simulink model "simli_gridSI"  (R2023b)
settings: Solver=VariableStepAuto  StartTime=0.0  StopTime=20  RelTol=1e-3
undefined symbols (not defined in the file or in its folder): c_f, Cbase1v, delta_vsc_0, G_dc_denom, G_dc_num, H_gen, H_vsm, Ibase_lv, k_d_vsm, k_p_p_vsm, k_p_q_vsm, ki_q, ki_vc, kp_vc, l_f, Lbase1v, M_gr_denom, M_gr_num, mppt_gain, omega_nom, omega_WTR_0, omega_WTR_n, P_aero_0, P_meas, Q_meas, r_f, r_grid, Rd, T_dc_denom, T_dc_num, Ts_power, v_D_t, v_Q_t, Vbase_lv, vect, x_sys, Zbase1v
libraries: slpidlib x2, spspowerguiLib x1
settings Model: Creator=Martin Pedersen  LastModifiedBy=marti

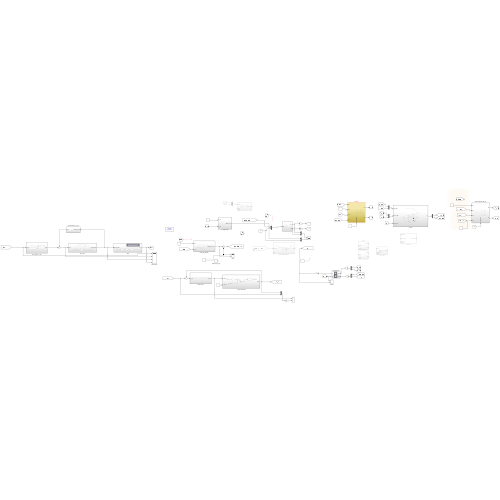
[thumbnail: Simulink's stored preview of the top-level diagram]
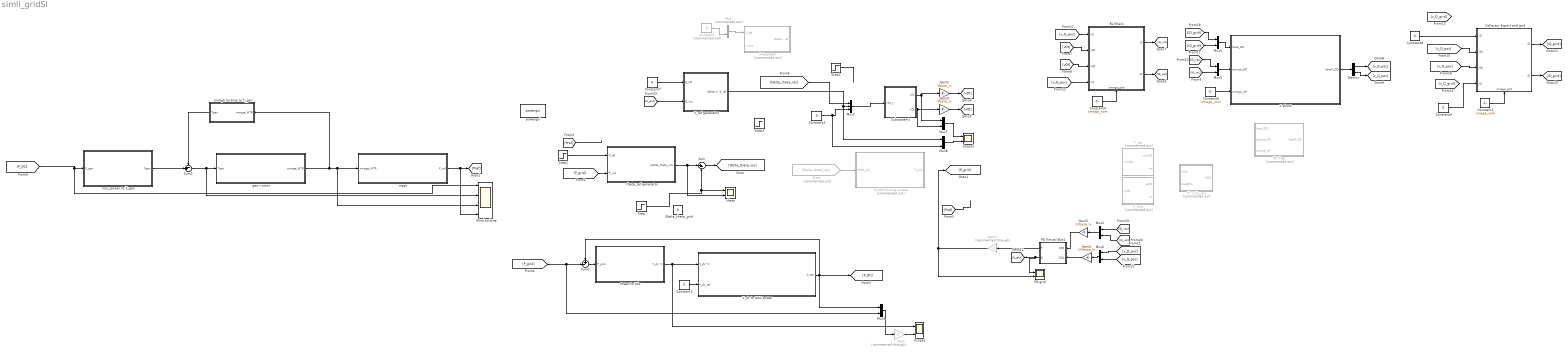
== system simli_gridSI ==
  C shunt : Subsystem
  Collector Export and grid : Subsystem
      settings: PortSchema="{\"entries\":[{\"content\":{\"sides\":[{\"content\":{\"connectorIds\":[\"In1\",\"In2\",\"In3\",\"In4\"]},\"type\":\"ConnectorPlacement.EquallySpacedRectSide\",\"uuid\":\"57ad71d1-5664-4b35-a20c-d71f7e1cdc47\"},{\"content\":{\"connectorIds\":[\"Out1\",\"Out2\"],\"side\":\"RIGHT\"},\"type\":\"ConnectorPlacement.EquallySpacedRectSide\",\"uuid\":\"8101605d-eedb-4c26-847d-0cc0ce629d60\"},{\"content\":{\"side\":\"TOP\"},\"type\":\"ConnectorPlacement.EquallySpacedRectSide\",\"uuid\":\"2627b00b-24a5-469a-be2d-9c3c8a1d2080\"},{\"content\":{\"connectorIds\":[\"In5\"],\"side\":\"BOTTOM\"},\"type\":\"ConnectorPlacement.EquallySpacedRectSide\",\"uuid\":\"fe553db7-7727-4a02-b1e7-5aedfb7840ee\"}]},\"type\":\"ConnectorPlacement.EquallySpacedConnector\",\"uuid\":\"f40200c8-ad5b-428c-8a4e-7641595b86c4\"}],\"packageUris\":[\"http://schema.mathworks.com/mf0/Connector/R2020b\"],\"version\":\"1.0\"}"
  Constant : Constant  Commented=on  Value=0
  Constant{1,3,7..9} (5 alike) : Constant  Value=0
  Constant2 : Constant  Value=omega_nom
  Constant4 : Constant  Value=omega_nom
  Constant5 : Constant  Value=omega_nom
  Demux : Demux  Outputs=2
  From : From  Commented=on  GotoTag=Delta_theta_vsc
  Gain : Gain  Commented=through  Gain=-1
  Gain1 : Gain  Commented=through  Gain=-1
  Gain2 : Gain  Gain=Vbase_lv
  Gain3 : Gain  Gain=Vbase_lv
  Gain4 : Gain  Gain=1/Vbase_lv
  Gain5 : Gain  Gain=1/Ibase_lv
  Mux : Mux  Commented=on  Inputs=2
  Mux{1,3..8} (7 alike) : Mux  Inputs=2
  Mux2 : Mux  Inputs=3
  PQ Virtual Bus1 : Subsystem
  PQ grid : Scope  NumInputPorts=2
  Power to Vdc : Subsystem
  RC filter : Subsystem  Commented=on  mask{Csource=c_f/omega_nom, Rd=0, VD0=1, VQ0=0}
      mask prompts: Csource "Net Capacitance"; Rd "Rdamp"
      mask help:
      | PI network, capacitance to enter is total.
      | Left and right current as input. Left and right voltage as output
      mask init:
      | inv_Csource=1/Csource;
      mask TypeOptions Csource: 8/Gain
      mask TypeOptions Rd: 1/Gain | 2/Gain
      mask TypeOptions VD0: VcpdR_int/InitialCondition
      mask TypeOptions VQ0: VcpqR_int/InitialCondition
  RL filter1 : Subsystem
      settings: PortSchema="{\"entries\":[{\"content\":{\"sides\":[{\"content\":{\"connectorIds\":[\"In1\",\"In2\",\"In3\",\"In4\"]},\"type\":\"ConnectorPlacement.EquallySpacedRectSide\",\"uuid\":\"57ad71d1-5664-4b35-a20c-d71f7e1cdc47\"},{\"content\":{\"connectorIds\":[\"Out1\",\"Out2\"],\"side\":\"RIGHT\"},\"type\":\"ConnectorPlacement.EquallySpacedRectSide\",\"uuid\":\"8101605d-eedb-4c26-847d-0cc0ce629d60\"},{\"content\":{\"side\":\"TOP\"},\"type\":\"ConnectorPlacement.EquallySpacedRectSide\",\"uuid\":\"2627b00b-24a5-469a-be2d-9c3c8a1d2080\"},{\"content\":{\"connectorIds\":[\"In5\"],\"side\":\"BOTTOM\"},\"type\":\"ConnectorPlacement.EquallySpacedRectSide\",\"uuid\":\"fe553db7-7727-4a02-b1e7-5aedfb7840ee\"}]},\"type\":\"ConnectorPlacement.EquallySpacedConnector\",\"uuid\":\"f40200c8-ad5b-428c-8a4e-7641595b86c4\"}],\"packageUris\":[\"http://schema.mathworks.com/mf0/Connector/R2020b\"],\"version\":\"1.0\"}"
  Scope1 : Scope  NumInputPorts=2
  Scope2 : Scope  NumInputPorts=2
  Step : Step  After=0.04  SampleTime=Ts_power
  Step1 : Step  After=0  SampleTime=Ts_power
  Step2 : Step  Time=5  After=0  SampleTime=Ts_power
  Step3 : Step  Time=5  After=0  SampleTime=Ts_power
  Subsystem : Subsystem  Commented=on
  Subsystem1 : Subsystem
  Sum : Sum  Inputs=|+-
  Sum1 : Sum  Inputs=+-|
  Sum2 : Sum  Inputs=-+|
  Synchronizing torque : Subsystem  Commented=on
  "T^{-1}_vsc" : Subsystem  Commented=on
  T_vsc : Subsystem  Commented=on  AncestorBlock=powerlib_meascontrol/Transformations/dq0 to Alpha-Beta-Zero/Subsystem1
  T_vsc1 : Subsystem  Commented=on  AncestorBlock=powerlib_meascontrol/Transformations/dq0 to Alpha-Beta-Zero/Subsystem1
  V_dc to MSC power : Subsystem
  V_ref generator : Subsystem
  Wind turbine : Scope  NumInputPorts=4
  \Delta_theta_grid : Constant  Value=0
  gen->rotor : Subsystem
  mppt : Subsystem
  msc_power to T_gen : Subsystem
  omega turbine to T_gen : Subsystem
  powergui : spspowerguiLib/powergui  Priority=1  SimulationMode=Discrete  SampleTime=Ts_power  frequency=60  Iterations=50  frequencyindice=60  Pbase=100e6  ErrMax=1e-4  UnitsV=kV  UnitsW=MW  buscounter=0  FunctionMessages=off  echomessages=off  EnableUseOfTLC=off  CurrentSourceSwitches=off  DisableSnubberDevices=off  DisableRonSwitches=off  DisableVfSwitches=off  DisplayEquations=off  AutomaticDiscreteSolvers=off  SolverType=Tustin/Backward Euler (TBE)  Interpol=off  ExternalGateDelay=off  methode=off  Ts=100  x0status=blocks  SPID=on  SwTol=0  HookPort=off  NonlinearTolerance=1e-4  nMaxIteration=100  ContinueOnMaxIteration=off  RestoreLinks=warning  ResistiveCurrentMeasurement=off  Frange=[0:2:500]  Ylog=off  Xlog=on  ShowGrid=off  save=off  variable=ZData  structure=0  ZoomFFT=off  StartTime=0.0  cycles=1  DisplayStyle=1  fundamental=60  FreqAxis=off  MaxFrequency=1000  frequencyindicesteady=1  RmsSteady=1  display=off
  theta : Scope  NumInputPorts=2
  theta_ref generator : Subsystem
  wires:
  theta_ref generator/1(\Delta_theta_vsm) -> theta/2, Sum/1
  Step/1 -> theta/1, Sum/2
  Sum/1 -> [Delta_theta_vsc]
  V_ref generator/1(\Delta V^d_ref) -> Mux8/1, Mux2/2
  Mux/1 -> Subsystem/1(V_ref)
  Constant/1 -> Mux/2
  From/1 -> Synchronizing torque/1(delta_vsc)
  PQ Virtual Bus1/1(P) -> Gain1/1
  [P_grid] -> theta_ref generator/2(P_vsc)
  [Pref] -> ?
  [Pref] -> ?
  gen->rotor/1(omega_WTR) -> omega turbine to T_gen/1(omega_WTR), Wind turbine/3, mppt/1(omega_WTR)
  Power to Vdc/1(V_dc^2) -> V_dc to MSC power/1(V_dc^2), Scope1/1
  V_dc to MSC power/1(P_DC) -> Mux1/1, [P_DC], Sum1/1
  Sum1/1 -> Power to Vdc/1(P_grid)
  [P_grid] -> Mux1/2, Sum1/2
  Mux1/1 -> Gain/1
  Sum2/1 -> Wind turbine/2, gen->rotor/1(Tgen)
  msc_power to T_gen/1(Tgen) -> Sum2/2
  omega turbine to T_gen/1(Tgen) -> Sum2/1
  [P_DC] -> Wind turbine/1, msc_power to T_gen/1(P_gen)
  mppt/1(P_ref) -> Wind turbine/4, [Pref]
  Constant1/1 -> V_dc to MSC power/2(V_dc_ref)
  Step1/1 -> theta_ref generator/1(P_ref)
  Gain/1 -> Scope1/2
  Constant3/1 -> Mux8/2, Mux2/3
  Step2/1 -> ?
  Mux2/1 -> Subsystem1/1(vdq_t)
  Constant4/1 -> RL filter1/5(omega_grid)
  Subsystem1/1(vDt) -> Mux7/1, Gain2/1
  Subsystem1/2(vQt) -> Mux7/2, Gain3/1
  [vDt] -> RL filter1/2(vDt)
  [vQt] -> RL filter1/3(vQt)
  Constant5/1 -> C shunt/3(omega_ref)
  RL filter1/2(iD) -> [iD_vsc]
  RL filter1/1(iQ) -> [iQ_vsc]
  Mux3/1 -> C shunt/2("Isource_DQ ")
  [iQ_vsc] -> Mux3/2
  [iD_vsc] -> Mux3/1
  C shunt/1(VpccR_DQ) -> Demux/1
  Demux/1 -> [v_D_poc]
  Demux/2 -> [v_Q_poc]
  [v_D_poc] -> RL filter1/1(vD)
  [v_Q_poc] -> RL filter1/4(vQ)
  Constant9/1 -> Collector Export and grid/4(vQ)
  Constant8/1 -> Collector Export and grid/1(vD)
  Collector Export and grid/1(iQ) -> [iQ_grid]
  Collector Export and grid/2(iD) -> [iD_grid]
  [v_Q_poc] -> Collector Export and grid/3(vQt)
  [v_D_poc] -> Collector Export and grid/2(vDt)
  Constant2/1 -> Collector Export and grid/5(omega_grid)
  Mux4/1 -> C shunt/1(Iload_DQ)
  [iQ_grid] -> Mux4/2
  [iD_grid] -> Mux4/1
  [iQ_vsc] -> Mux5/2
  [iD_vsc] -> Mux5/1
  Mux5/1 -> Gain5/1
  [v_Q_poc] -> Mux6/2
  [v_D_poc] -> Mux6/1
  Mux6/1 -> Gain4/1
  PQ Virtual Bus1/2(Q) -> PQ grid/1, [Q_grid]
  [Q_grid] -> V_ref generator/2(Q_vsc)
  Constant7/1 -> V_ref generator/1(Q_ref)
  Mux7/1 -> Scope2/1
  Mux8/1 -> Scope2/2
  [Delta_theta_vsc] -> Mux2/1
  Gain1/1 -> [P_grid], PQ grid/2
  Gain2/1 -> [vDt]
  Gain3/1 -> [vQt]
  Gain4/1 -> PQ Virtual Bus1/2(VDQ)
  Gain5/1 -> PQ Virtual Bus1/1(IDQ)

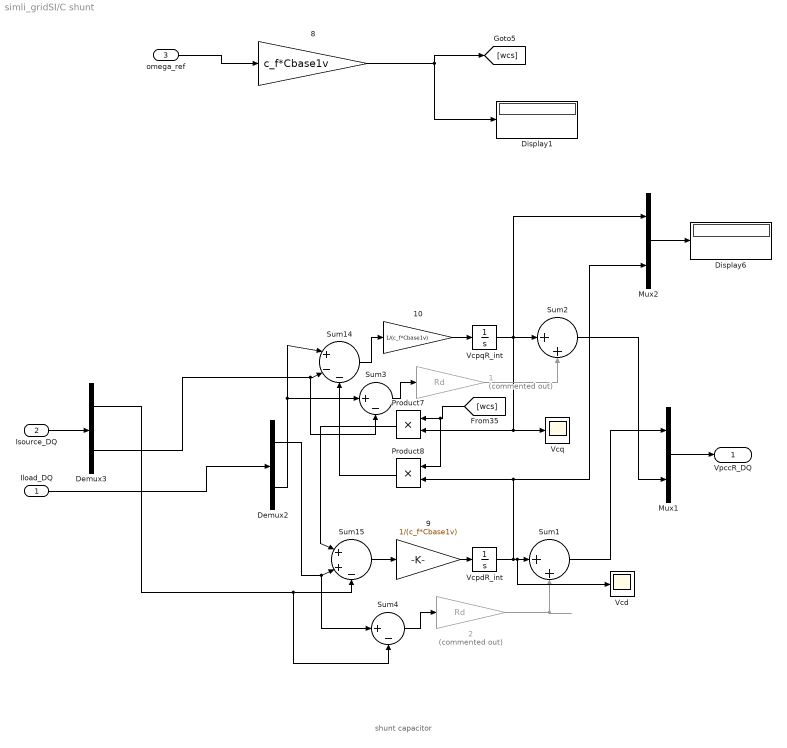
== system simli_gridSI/C shunt ==
  note: shunt capacitor
  Iload_DQ : Inport
  "Isource_DQ " : Inport  Port=2
  omega_ref : Inport  Port=3
  1 : Gain  Commented=on  Gain=Rd
  10 : Gain  Gain=1/(c_f*Cbase1v)
  2 : Gain  Commented=on  Gain=Rd
  8 : Gain  Gain=c_f*Cbase1v
  9 : Gain  Gain=1/(c_f*Cbase1v)
  Demux2 : Demux  Outputs=2
  Demux3 : Demux  Outputs=2
  Display1 : Display
  Display6 : Display
  Mux1 : Mux  Inputs=2
  Mux2 : Mux  Inputs=2
  Product7 : Product
  Product8 : Product
  Sum1 : Sum  Inputs=|++
  Sum14 : Sum  Inputs=|+--
  Sum15 : Sum  Inputs=|++-
  Sum2 : Sum  Inputs=|++
  Sum3 : Sum  Inputs=|+-
  Sum4 : Sum  Inputs=|+-
  Vcd : Scope
  VcpdR_int : Integrator  UpperSaturationLimit=50  LowerSaturationLimit=-1000
  VcpqR_int : Integrator  UpperSaturationLimit=50  LowerSaturationLimit=-1000
  Vcq : Scope
  VpccR_DQ : Outport  VectorParamsAs1DForOutWhenUnconnected=off
  wires:
  Mux1/1 -> VpccR_DQ/1
  Demux2/1 -> Sum15/2, Sum4/1
  VcpqR_int/1 -> Vcq/1, Product7/2, Sum2/1, Mux2/1
  1/1 -> Sum2/2
  2/1 -> Sum1/2
  Sum15/1 -> 9/1
  Product8/1 -> Sum14/3
  Sum14/1 -> 10/1
  8/1 -> [wcs], Display1/1
  Demux3/1 -> Sum15/3, Sum4/2
  "Isource_DQ "/1 -> Demux3/1
  Product7/1 -> Sum15/1
  omega_ref/1 -> 8/1
  Demux2/2 -> Sum14/1, Sum3/1
  [wcs] -> Product8/1, Product7/1
  Iload_DQ/1 -> Demux2/1
  9/1 -> VcpdR_int/1
  Demux3/2 -> Sum14/2, Sum3/2
  Sum3/1 -> 1/1
  10/1 -> VcpqR_int/1
  Mux2/1 -> Display6/1
  Sum4/1 -> 2/1
  Sum1/1 -> Mux1/1
  Sum2/1 -> Mux1/2
  VcpdR_int/1 -> Vcd/1, Sum1/1, Product8/2, Mux2/2

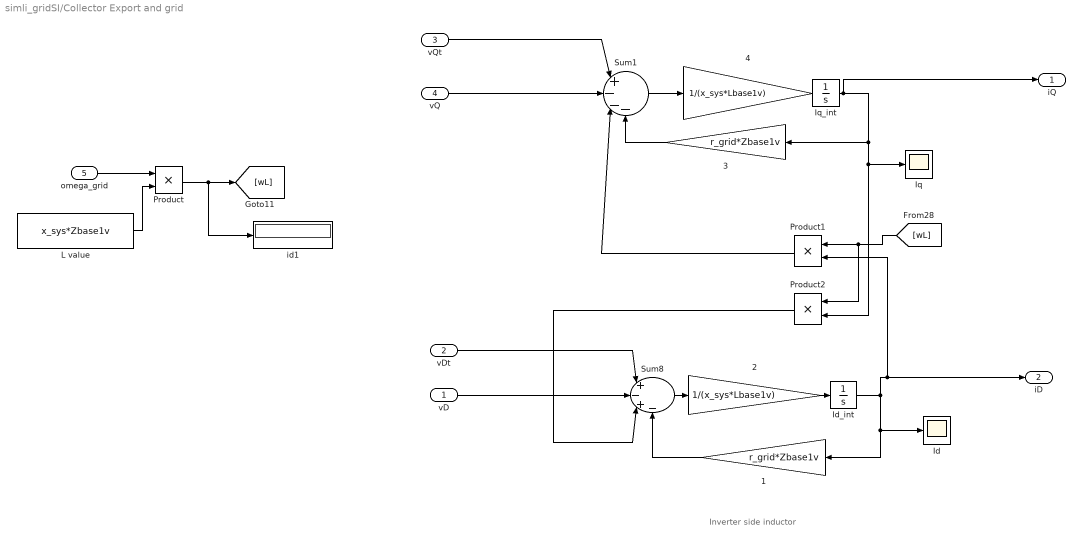
== system simli_gridSI/Collector Export and grid ==
  note: Inverter side inductor
  vD : Inport
  vDt : Inport  Port=2
  vQt : Inport  Port=3
  vQ : Inport  Port=4
  omega_grid : Inport  Port=5
  1 : Gain  Gain=r_grid*Zbase1v
  2 : Gain  Gain=1/(x_sys*Lbase1v)
  3 : Gain  Gain=r_grid*Zbase1v
  4 : Gain  Gain=1/(x_sys*Lbase1v)
  Id : Scope
  Id_int : Integrator  UpperSaturationLimit=50  LowerSaturationLimit=-1000
  Iq : Scope
  Iq_int : Integrator  UpperSaturationLimit=50  LowerSaturationLimit=-1000
  L value : Constant  Value=x_sys*Zbase1v  SampleTime=-1
  Product : Product
  Product1 : Product
  Product2 : Product
  Sum1 : Sum  Inputs=|+---
  Sum8 : Sum  Inputs=|+-+-
  id1 : Display
  iQ : Outport
  iD : Outport  Port=2
  wires:
  [wL] -> Product2/1, Product1/1
  Id_int/1 -> 1/1, Id/1, iD/1, Product1/2
  1/1 -> Sum8/4
  Product1/1 -> Sum1/3
  3/1 -> Sum1/4
  Sum1/1 -> 4/1
  2/1 -> Id_int/1
  Sum8/1 -> 2/1
  4/1 -> Iq_int/1
  Iq_int/1 -> iQ/1, Product2/2, Iq/1, 3/1
  Product2/1 -> Sum8/3
  vDt/1 -> Sum8/1
  vD/1 -> Sum8/2
  vQt/1 -> Sum1/1
  vQ/1 -> Sum1/2
  L value/1 -> Product/2
  Product/1 -> id1/1, [wL]
  omega_grid/1 -> Product/1

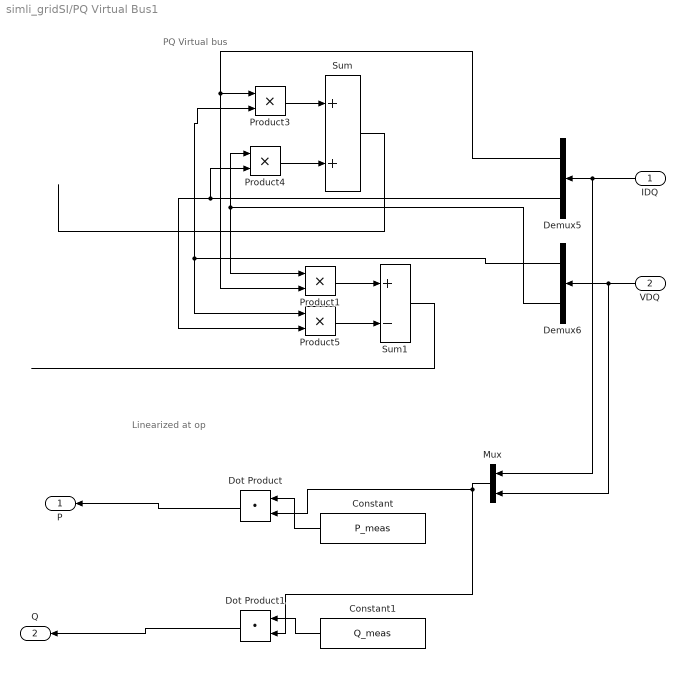
== system simli_gridSI/PQ Virtual Bus1 ==
  note: Linearized at op
  note: PQ Virtual bus
  IDQ : Inport
  VDQ : Inport  Port=2
  Constant : Constant  Value=P_meas
  Constant1 : Constant  Value=Q_meas
  Demux5 : Demux  Outputs=[vect vect]
  Demux6 : Demux  Outputs=[vect vect]
  Dot Product : DotProduct  OutDataTypeStr=Inherit: Inherit via internal rule
  Dot Product1 : DotProduct  OutDataTypeStr=Inherit: Inherit via internal rule
  Mux : Mux  Inputs=2
  Product{1,3..5} (4 alike) : Product  InputSameDT=on  SaturateOnIntegerOverflow=on  OutDataTypeStr=Inherit: Same as first input
  Sum : Sum  InputSameDT=on  SaturateOnIntegerOverflow=on  OutDataTypeStr=Inherit: Same as first input
  Sum1 : Sum  Inputs=+-  InputSameDT=on  SaturateOnIntegerOverflow=on  OutDataTypeStr=Inherit: Same as first input
  P : Outport
  Q : Outport  Port=2
  wires:
  Sum/1 -> ?
  VDQ/1 -> Mux/2, Demux6/1
  IDQ/1 -> Mux/1, Demux5/1
  Sum1/1 -> ?
  Product5/1 -> Sum1/2
  Product1/1 -> Sum1/1
  Demux6/2 -> Product4/1, Product1/1
  Demux5/1 -> Product1/2, Product3/1
  Demux6/1 -> Product3/2, Product5/1
  Product4/1 -> Sum/2
  Demux5/2 -> Product5/2, Product4/2
  Product3/1 -> Sum/1
  Constant/1 -> Dot Product/1
  Mux/1 -> Dot Product1/2, Dot Product/2
  Constant1/1 -> Dot Product1/1
  Dot Product1/1 -> Q/1
  Dot Product/1 -> P/1

== system simli_gridSI/Power to Vdc ==
  P_grid : Inport
  DC dynamics : TransferFcn  Numerator=T_dc_num{1}  Denominator=T_dc_denom{1}
  msc current control : TransferFcn  Commented=through  Denominator=[0.01 1]
  V_dc^2 : Outport
  wires:
  P_grid/1 -> msc current control/1
  DC dynamics/1 -> V_dc^2/1
  msc current control/1 -> DC dynamics/1

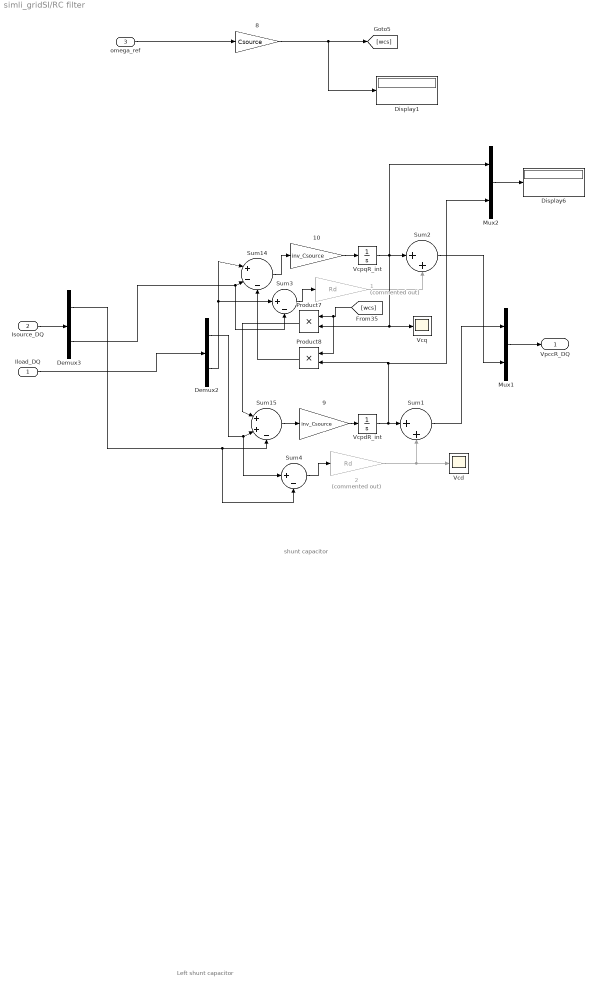
== system simli_gridSI/RC filter ==
  note: shunt capacitor
  note: Left shunt capacitor
  Iload_DQ : Inport
  "Isource_DQ " : Inport  Port=2
  omega_ref : Inport  Port=3
  1 : Gain  Commented=on  Gain=Rd
  10 : Gain  Gain=inv_Csource
  2 : Gain  Commented=on  Gain=Rd
  8 : Gain  Gain=Csource
  9 : Gain  Gain=inv_Csource
  Demux2 : Demux  Outputs=2
  Demux3 : Demux  Outputs=2
  Display1 : Display
  Display6 : Display
  Mux1 : Mux  Inputs=2
  Mux2 : Mux  Inputs=2
  Product7 : Product
  Product8 : Product
  Sum1 : Sum  Inputs=|++
  Sum14 : Sum  Inputs=|+--
  Sum15 : Sum  Inputs=|++-
  Sum2 : Sum  Inputs=|++
  Sum3 : Sum  Inputs=|+-
  Sum4 : Sum  Inputs=|+-
  Vcd : Scope
  VcpdR_int : Integrator  InitialCondition=VD0  UpperSaturationLimit=50  LowerSaturationLimit=-1000
  VcpqR_int : Integrator  InitialCondition=VQ0  UpperSaturationLimit=50  LowerSaturationLimit=-1000
  Vcq : Scope
  VpccR_DQ : Outport  VectorParamsAs1DForOutWhenUnconnected=off
  wires:
  Sum4/1 -> 2/1
  Sum3/1 -> 1/1
  Mux2/1 -> Display6/1
  2/1 -> Vcd/1, Sum1/2
  1/1 -> Sum2/2
  Sum2/1 -> Mux1/2
  Sum1/1 -> Mux1/1
  VcpdR_int/1 -> Sum1/1, Product8/2, Mux2/2
  Demux3/1 -> Sum15/3, Sum4/2
  Demux3/2 -> Sum14/2, Sum3/2
  "Isource_DQ "/1 -> Demux3/1
  Iload_DQ/1 -> Demux2/1
  Demux2/2 -> Sum14/1, Sum3/1
  Demux2/1 -> Sum15/2, Sum4/1
  9/1 -> VcpdR_int/1
  Sum14/1 -> 10/1
  [wcs] -> Product8/1, Product7/1
  VcpqR_int/1 -> Vcq/1, Product7/2, Sum2/1, Mux2/1
  Product7/1 -> Sum15/1
  10/1 -> VcpqR_int/1
  Sum15/1 -> 9/1
  Product8/1 -> Sum14/3
  Mux1/1 -> VpccR_DQ/1
  8/1 -> Display1/1, [wcs]
  omega_ref/1 -> 8/1

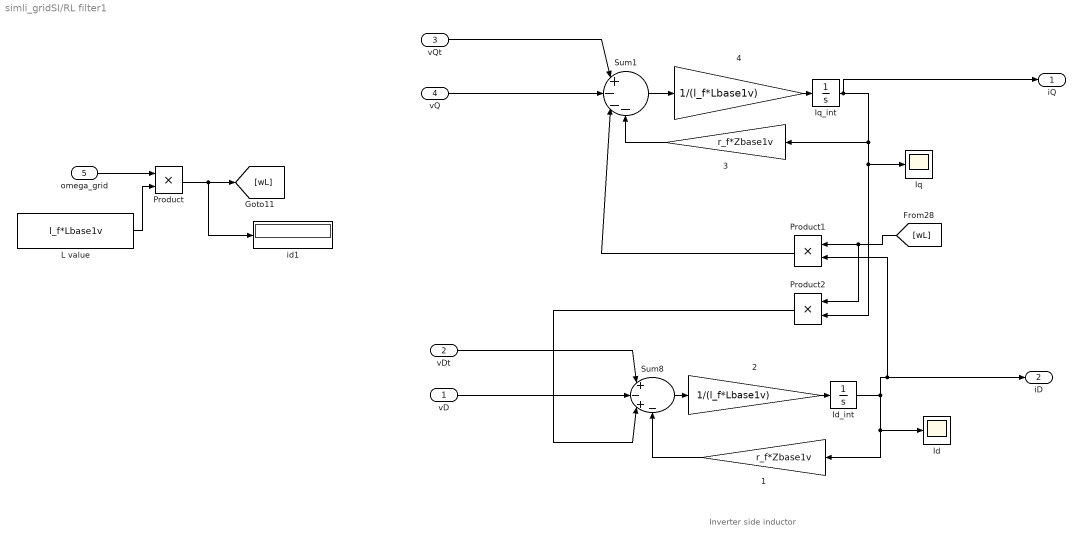
== system simli_gridSI/RL filter1 ==
  note: Inverter side inductor
  vD : Inport
  vDt : Inport  Port=2
  vQt : Inport  Port=3
  vQ : Inport  Port=4
  omega_grid : Inport  Port=5
  1 : Gain  Gain=r_f*Zbase1v
  2 : Gain  Gain=1/(l_f*Lbase1v)
  3 : Gain  Gain=r_f*Zbase1v
  4 : Gain  Gain=1/(l_f*Lbase1v)
  Id : Scope
  Id_int : Integrator  UpperSaturationLimit=50  LowerSaturationLimit=-1000
  Iq : Scope
  Iq_int : Integrator  UpperSaturationLimit=50  LowerSaturationLimit=-1000
  L value : Constant  Value=l_f*Lbase1v  SampleTime=-1
  Product : Product
  Product1 : Product
  Product2 : Product
  Sum1 : Sum  Inputs=|+---
  Sum8 : Sum  Inputs=|+-+-
  id1 : Display
  iQ : Outport
  iD : Outport  Port=2
  wires:
  omega_grid/1 -> Product/1
  Product/1 -> [wL], id1/1
  L value/1 -> Product/2
  vQ/1 -> Sum1/2
  vQt/1 -> Sum1/1
  vD/1 -> Sum8/2
  vDt/1 -> Sum8/1
  Product2/1 -> Sum8/3
  Iq_int/1 -> 3/1, Iq/1, Product2/2, iQ/1
  4/1 -> Iq_int/1
  Sum8/1 -> 2/1
  2/1 -> Id_int/1
  Sum1/1 -> 4/1
  3/1 -> Sum1/4
  Product1/1 -> Sum1/3
  1/1 -> Sum8/4
  Id_int/1 -> Product1/2, iD/1, Id/1, 1/1
  [wL] -> Product1/1, Product2/1

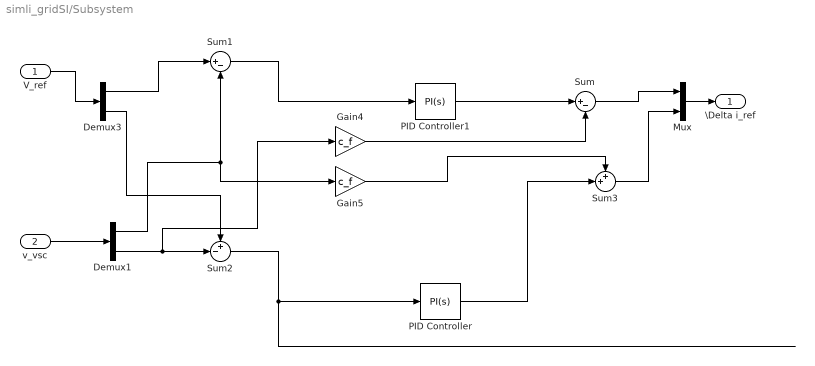
== system simli_gridSI/Subsystem ==
  V_ref : Inport
  v_vsc : Inport  Port=2
  Demux1 : Demux  Outputs=[vect vect]
  Demux3 : Demux  Outputs=[vect vect]
  Gain4 : Gain  Gain=c_f
  Gain5 : Gain  Gain=c_f
  Mux : Mux  Inputs=2
  PID Controller : slpidlib/PID Controller  Controller=PI  Form=Parallel  TimeDomain=Continuous-time  UseExternalTs=off  SampleTime=-1  IntegratorMethod=Forward Euler  FilterMethod=Forward Euler  ControllerParametersSource=internal  P=kp_vc  I=ki_vc  UseKiTs=off  D=0  N=100  UseFilter=on  TunerSelectOption=Transfer Function Based (PID Tuner App)  InitialConditionSource=internal  InitialConditionForIntegrator=0  InitialConditionForFilter=0  DifferentiatorICPrevScaledInput=0  ExternalReset=none  TrackingMode=off  Kt=1  LimitOutput=off  SatLimitsSource=internal  UpperSaturationLimit=2  LowerSaturationLimit=-2  LinearizeAsGain=off  AntiWindupMode=none  Kb=1  LimitIntegrator=off  UpperIntegratorSaturationLimit=inf  LowerIntegratorSaturationLimit=-inf  POutMin=[]  POutMax=[]  IOutMin=[]  IOutMax=[]  DOutMin=[]  DOutMax=[]  NOutMin=[]  NOutMax=[]  SumOutMin=[]  SumOutMax=[]  SaturationOutMin=[]  SaturationOutMax=[]  PParamMin=[]  PParamMax=[]  IParamMin=[]  IParamMax=[]  DParamMin=[]  DParamMax=[]  NParamMin=[]  NParamMax=[]  KbParamMin=[]  KbParamMax=[]  KtParamMin=[]  KtParamMax=[]  KbOutMin=[]  KbOutMax=[]  KtOutMin=[]  KtOutMax=[]  IntegratorOutMin=[]  IntegratorOutMax=[]  FilterOutMin=[]  FilterOutMax=[]  SumI1OutMin=[]  SumI1OutMax=[]  SumI2OutMin=[]  SumI2OutMax=[]  SumI3OutMin=[]  SumI3OutMax=[]  SumI4OutMin=[]  SumI4OutMax=[]  SumDOutMin=[]  SumDOutMax=[]  DifferentiatorOutMin=[]  DifferentiatorOutMax=[]  FilterDiffOutCoefMin=[]  FilterDiffOutCoefMax=[]  ReciprocalOutMin=[]  ReciprocalOutMax=[]  SumDenOutMin=[]  SumDenOutMax=[]  SumNumOutMin=[]  SumNumOutMax=[]  DivideOutMin=[]  DivideOutMax=[]  UdiffTsProdOutMin=[]  UdiffTsProdOutMax=[]  NTsProdOutMin=[]  NTsProdOutMax=[]  UintegralTsProdOutMin=[]  UintegralTsProdOutMax=[]  UngainTsProdOutMin=[]  UngainTsProdOutMax=[]  ClampingZeroOutDataTypeStr=Inherit: Inherit via back propagation  ClampingZeroOutMin=[]  ClampingZeroOutMax=[]  FilterDenConstantOutDataTypeStr=Inherit: Inherit via back propagation  FilterDenConstantOutMin=[]  FilterDenConstantOutMax=[]  PCopyOutDataTypeStr=Inherit: Inherit via back propagation  PCopyOutMin=[]  PCopyOutMax=[]  NCopyOutDataTypeStr=Inherit: Inherit via back propagation  NCopyOutMin=[]  NCopyOutMax=[]  IntegratorContinuousStateAttributes=''  IntegratorStateMustResolveToSignalObject=off  IntegratorRTWStateStorageClass=Auto  FilterContinuousStateAttributes=''  FilterStateMustResolveToSignalObject=off  FilterRTWStateStorageClass=Auto  ParallelPVariant=InternalParameters  IdealPVariant=Disabled  IVariant=InternalParameters  DVariant=Disabled  IntegratorVariant=Continuous  SatVariant=Disabled  AWVariant=Passthrough  PCopyVariant=Disabled  TRVariant=Disabled  FdbkBlocksVariant=Forward  IdealPFdbkVariant=Disabled  SatFdbkVariant=Disabled  DerivativeFilterVariant=Disabled  NVariant=Disabled  NCopyVariant=Disabled_SignalSpec  FilterICVariant=Disabled  IntegratorICVariant=InternalICs  ExternalResetVariant=Disabled  TRSumVariant=Passthrough  SumFdbkVariant=Disabled  SumVariant=Sum_PI  TsampFilterVariant=InternalTs  TsampNgainVariant=Passthrough  TsampIntegralVariant=Disabled_SignalSpec  ExternalSaturationOutDataTypeStr=Inherit: Same as second input
  PID Controller1 : slpidlib/PID Controller  Controller=PI  Form=Parallel  TimeDomain=Continuous-time  UseExternalTs=off  SampleTime=-1  IntegratorMethod=Forward Euler  FilterMethod=Forward Euler  ControllerParametersSource=internal  P=kp_vc  I=ki_vc  UseKiTs=off  D=0  N=100  UseFilter=on  TunerSelectOption=Transfer Function Based (PID Tuner App)  InitialConditionSource=internal  InitialConditionForIntegrator=1  InitialConditionForFilter=0  DifferentiatorICPrevScaledInput=0  ExternalReset=none  TrackingMode=off  Kt=1  LimitOutput=off  SatLimitsSource=internal  UpperSaturationLimit=2  LowerSaturationLimit=-2  LinearizeAsGain=off  AntiWindupMode=none  Kb=1  LimitIntegrator=off  UpperIntegratorSaturationLimit=inf  LowerIntegratorSaturationLimit=-inf  POutMin=[]  POutMax=[]  IOutMin=[]  IOutMax=[]  DOutMin=[]  DOutMax=[]  NOutMin=[]  NOutMax=[]  SumOutMin=[]  SumOutMax=[]  SaturationOutMin=[]  SaturationOutMax=[]  PParamMin=[]  PParamMax=[]  IParamMin=[]  IParamMax=[]  DParamMin=[]  DParamMax=[]  NParamMin=[]  NParamMax=[]  KbParamMin=[]  KbParamMax=[]  KtParamMin=[]  KtParamMax=[]  KbOutMin=[]  KbOutMax=[]  KtOutMin=[]  KtOutMax=[]  IntegratorOutMin=[]  IntegratorOutMax=[]  FilterOutMin=[]  FilterOutMax=[]  SumI1OutMin=[]  SumI1OutMax=[]  SumI2OutMin=[]  SumI2OutMax=[]  SumI3OutMin=[]  SumI3OutMax=[]  SumI4OutMin=[]  SumI4OutMax=[]  SumDOutMin=[]  SumDOutMax=[]  DifferentiatorOutMin=[]  DifferentiatorOutMax=[]  FilterDiffOutCoefMin=[]  FilterDiffOutCoefMax=[]  ReciprocalOutMin=[]  ReciprocalOutMax=[]  SumDenOutMin=[]  SumDenOutMax=[]  SumNumOutMin=[]  SumNumOutMax=[]  DivideOutMin=[]  DivideOutMax=[]  UdiffTsProdOutMin=[]  UdiffTsProdOutMax=[]  NTsProdOutMin=[]  NTsProdOutMax=[]  UintegralTsProdOutMin=[]  UintegralTsProdOutMax=[]  UngainTsProdOutMin=[]  UngainTsProdOutMax=[]  ClampingZeroOutDataTypeStr=Inherit: Inherit via back propagation  ClampingZeroOutMin=[]  ClampingZeroOutMax=[]  FilterDenConstantOutDataTypeStr=Inherit: Inherit via back propagation  FilterDenConstantOutMin=[]  FilterDenConstantOutMax=[]  PCopyOutDataTypeStr=Inherit: Inherit via back propagation  PCopyOutMin=[]  PCopyOutMax=[]  NCopyOutDataTypeStr=Inherit: Inherit via back propagation  NCopyOutMin=[]  NCopyOutMax=[]  IntegratorContinuousStateAttributes=''  IntegratorStateMustResolveToSignalObject=off  IntegratorRTWStateStorageClass=Auto  FilterContinuousStateAttributes=''  FilterStateMustResolveToSignalObject=off  FilterRTWStateStorageClass=Auto  ParallelPVariant=InternalParameters  IdealPVariant=Disabled  IVariant=InternalParameters  DVariant=Disabled  IntegratorVariant=Continuous  SatVariant=Disabled  AWVariant=Passthrough  PCopyVariant=Disabled  TRVariant=Disabled  FdbkBlocksVariant=Forward  IdealPFdbkVariant=Disabled  SatFdbkVariant=Disabled  DerivativeFilterVariant=Disabled  NVariant=Disabled  NCopyVariant=Disabled_SignalSpec  FilterICVariant=Disabled  IntegratorICVariant=InternalICs  ExternalResetVariant=Disabled  TRSumVariant=Passthrough  SumFdbkVariant=Disabled  SumVariant=Sum_PI  TsampFilterVariant=InternalTs  TsampNgainVariant=Passthrough  TsampIntegralVariant=Disabled_SignalSpec  ExternalSaturationOutDataTypeStr=Inherit: Same as second input
  Sum : Sum  Inputs=|+-
  Sum1 : Sum  Inputs=|+-
  Sum2 : Sum  Inputs=+-|
  Sum3 : Sum  Inputs=++|
  \Delta i_ref : Outport
  wires:
  Demux1/1 -> Sum1/2, Gain5/1
  Demux3/1 -> Sum1/1
  Sum2/1 -> PID Controller/1
  Demux1/2 -> Gain4/1, Sum2/2
  PID Controller/1 -> Sum3/2
  v_vsc/1 -> Demux1/1
  Gain4/1 -> Sum/2
  V_ref/1 -> Demux3/1
  Demux3/2 -> Sum2/1
  Sum1/1 -> PID Controller1/1
  Gain5/1 -> Sum3/1
  PID Controller1/1 -> Sum/1
  Mux/1 -> \Delta i_ref/1
  Sum/1 -> Mux/1
  Sum3/1 -> Mux/2

== system simli_gridSI/Subsystem1 ==
  vdq_t : Inport
  Constant : Constant  Value=v_D_t
  Constant1 : Constant  Value=v_Q_t
  Dot Product : DotProduct  OutDataTypeStr=Inherit: Inherit via internal rule
  Dot Product1 : DotProduct  OutDataTypeStr=Inherit: Inherit via internal rule
  Gain1 : Gain  Gain=v_D_t
  Gain2 : Gain  Gain=v_Q_t
  vDt : Outport
  vQt : Outport  Port=2
  wires:
  Dot Product/1 -> vDt/1
  vdq_t/1 -> Dot Product/1, Dot Product1/1
  Dot Product1/1 -> vQt/1
  Constant/1 -> Dot Product/2
  Constant1/1 -> Dot Product1/2

== system simli_gridSI/Synchronizing torque ==
  delta_vsc : Inport
  Constant : Constant  Value=1/x_sys
  Constant1 : Constant  Value=cos(delta_vsc_0)
  Product : Product  Inputs=3
  P_grid : Outport
  wires:
  delta_vsc/1 -> Product/1
  Product/1 -> P_grid/1
  Constant/1 -> Product/2
  Constant1/1 -> Product/3

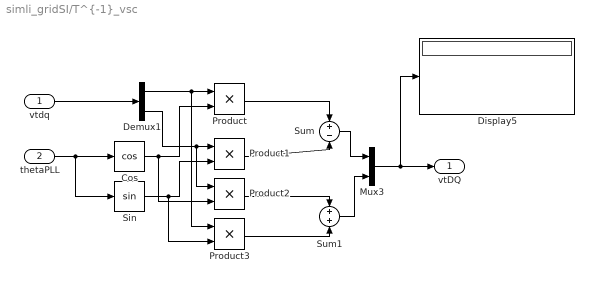
== system simli_gridSI/T^{-1}_vsc ==
  vtdq : Inport
  thetaPLL : Inport  Port=2
  Cos : Trigonometry  Operator=cos
  Demux1 : Demux  Outputs=2
  Display5 : Display
  Mux3 : Mux  Inputs=2
  Product{,1..3} (4 alike) : Product
  Sin : Trigonometry
  Sum : Sum  Inputs=+-
  Sum1 : Sum
  vtDQ : Outport  InitialOutput=[0,0]  VectorParamsAs1DForOutWhenUnconnected=off
  wires:
  Product3/1 -> Sum1/2
  Sum1/1 -> Mux3/2
  Demux1/1 -> Product3/1, Product/1
  vtdq/1 -> Demux1/1
  Demux1/2 -> Product2/1, Product1/1
  Sin/1 -> Product3/2, Product1/2
  Product2/1 -> Sum1/1
  Cos/1 -> Product2/2, Product/2
  Mux3/1 -> vtDQ/1, Display5/1
  thetaPLL/1 -> Cos/1, Sin/1
  Sum/1 -> Mux3/1
  Product/1 -> Sum/1
  Product1/1 -> Sum/2

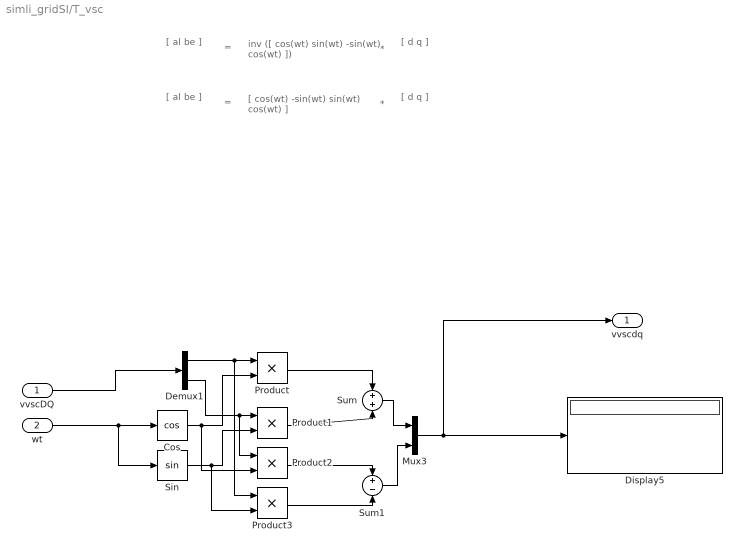
== system simli_gridSI/T_vsc ==
  note: *
  note: =
  note: inv ([  cos(wt)   sin(wt)
      |    -sin(wt)    cos(wt)   ])
  note: [ d
      |    q ]
  note: [  al
      |     be  ]
  note: *
  note: =
  note: [  cos(wt)   -sin(wt)
      |    sin(wt)    cos(wt)   ]
  note: [ d
      |    q ]
  note: [  al
      |     be  ]
  vvscDQ : Inport
  wt : Inport  Port=2
  Cos : Trigonometry  Operator=cos
  Demux1 : Demux  Outputs=2
  Display5 : Display
  Mux3 : Mux  Inputs=2
  Product{,1..3} (4 alike) : Product
  Sin : Trigonometry
  Sum : Sum
  Sum1 : Sum  Inputs=+-
  vvscdq : Outport  InitialOutput=[0,0]  VectorParamsAs1DForOutWhenUnconnected=off
  wires:
  Demux1/1 -> Product/1, Product3/1
  wt/1 -> Sin/1, Cos/1
  Product/1 -> Sum/1
  Sum/1 -> Mux3/1
  Mux3/1 -> Display5/1, vvscdq/1
  Sum1/1 -> Mux3/2
  vvscDQ/1 -> Demux1/1
  Sin/1 -> Product1/2, Product3/2
  Product1/1 -> Sum/2
  Cos/1 -> Product/2, Product2/2
  Product2/1 -> Sum1/1
  Demux1/2 -> Product1/1, Product2/1
  Product3/1 -> Sum1/2

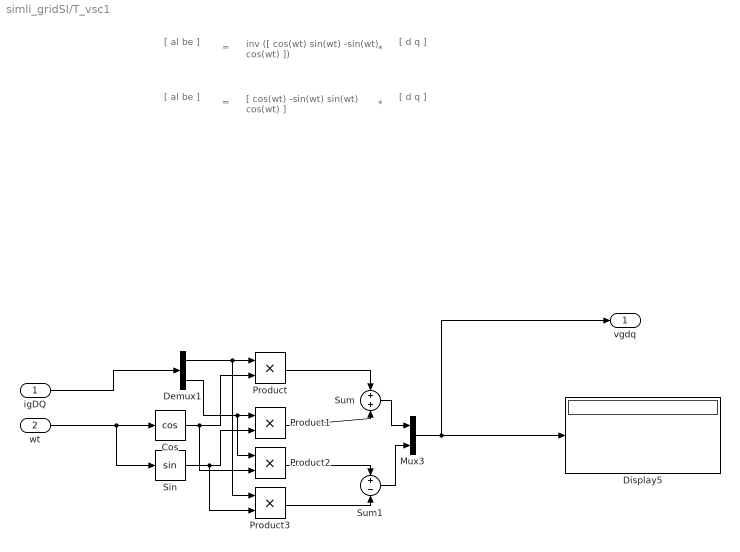
== system simli_gridSI/T_vsc1 ==
  note: [  al
      |     be  ]
  note: [ d
      |    q ]
  note: [  cos(wt)   -sin(wt)
      |    sin(wt)    cos(wt)   ]
  note: =
  note: *
  note: [  al
      |     be  ]
  note: [ d
      |    q ]
  note: inv ([  cos(wt)   sin(wt)
      |    -sin(wt)    cos(wt)   ])
  note: =
  note: *
  igDQ : Inport
  wt : Inport  Port=2
  Cos : Trigonometry  Operator=cos
  Demux1 : Demux  Outputs=2
  Display5 : Display
  Mux3 : Mux  Inputs=2
  Product{,1..3} (4 alike) : Product
  Sin : Trigonometry
  Sum : Sum
  Sum1 : Sum  Inputs=+-
  vgdq : Outport  InitialOutput=[0,0]  VectorParamsAs1DForOutWhenUnconnected=off
  wires:
  Product3/1 -> Sum1/2
  Demux1/2 -> Product2/1, Product1/1
  Product2/1 -> Sum1/1
  Cos/1 -> Product2/2, Product/2
  Product1/1 -> Sum/2
  Sin/1 -> Product3/2, Product1/2
  igDQ/1 -> Demux1/1
  Sum1/1 -> Mux3/2
  Mux3/1 -> vgdq/1, Display5/1
  Sum/1 -> Mux3/1
  Product/1 -> Sum/1
  wt/1 -> Cos/1, Sin/1
  Demux1/1 -> Product3/1, Product/1

== system simli_gridSI/V_dc to MSC power ==
  V_dc^2 : Inport
  V_dc_ref : Inport  Port=2
  G_dc : TransferFcn  Numerator=G_dc_num{1}  Denominator=G_dc_denom{1}
  Gain : Gain
  Square : Math  Commented=through  Operator=square
  Square1 : Math  Commented=through  Operator=square
  Sum : Sum  Inputs=|-+
  P_DC : Outport
  wires:
  V_dc^2/1 -> Square/1
  G_dc/1 -> P_DC/1
  Sum/1 -> Gain/1
  V_dc_ref/1 -> Square1/1
  Square/1 -> Sum/1
  Square1/1 -> Sum/2
  Gain/1 -> G_dc/1

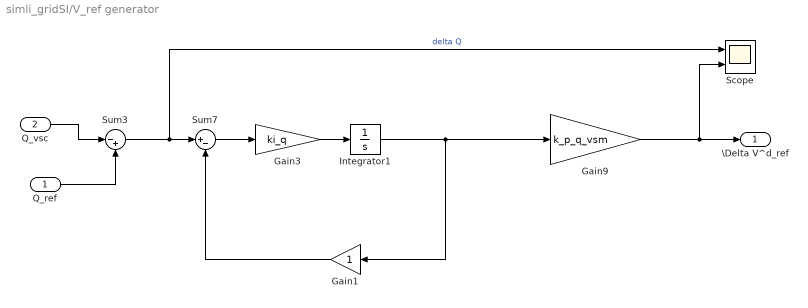
== system simli_gridSI/V_ref generator ==
  Q_ref : Inport
  Q_vsc : Inport  Port=2
  Gain1 : Gain
  Gain3 : Gain  Gain=ki_q
  Gain9 : Gain  Gain=k_p_q_vsm
  Integrator1 : Integrator
  Scope : Scope  NumInputPorts=2
  Sum3 : Sum  Inputs=|-+
  Sum7 : Sum  Inputs=|+-
  \Delta V^d_ref : Outport
  wires:
  Gain9/1 -> Scope/2, \Delta V^d_ref/1
  Integrator1/1 -> Gain9/1, Gain1/1
  Gain1/1 -> Sum7/2
  Gain3/1 -> Integrator1/1
  Sum7/1 -> Gain3/1
  Q_ref/1 -> Sum3/2
  Q_vsc/1 -> Sum3/1
  Sum3/1 -> Scope/1, Sum7/1  "delta Q"

== system simli_gridSI/gen->rotor ==
  Tgen : Inport
  Gain : Gain  Gain=1/(2*H_gen)
  Integrator : Integrator
  Sum : Sum  Inputs=+-|
  Transfer Fcn : TransferFcn  Numerator=M_gr_num{1}  Denominator=M_gr_denom{1}
  omega_WTR : Outport
  wires:
  Sum/1 -> Gain/1
  Gain/1 -> Integrator/1
  Integrator/1 -> Transfer Fcn/1, omega_WTR/1
  Tgen/1 -> Sum/2
  Transfer Fcn/1 -> Sum/1

== system simli_gridSI/mppt ==
  note: Remember to add SI->PU conversion before output
  omega_WTR : Inport
  Gain : Gain  Gain=omega_WTR_n
  Gain1 : Gain  Gain=1/(15e6)
  MPPT_GAIN : Gain  Gain=mppt_gain
  P_ref : Outport
  wires:
  omega_WTR/1 -> Gain/1
  MPPT_GAIN/1 -> Gain1/1
  Gain/1 -> MPPT_GAIN/1
  Gain1/1 -> P_ref/1

== system simli_gridSI/msc_power to T_gen ==
  P_gen : Inport
  Divide : Product  Inputs=*/
  turbine omega operating point : Constant  Value=(omega_WTR_0/omega_WTR_n)
  Tgen : Outport
  wires:
  P_gen/1 -> Divide/1
  turbine omega operating point/1 -> Divide/2
  Divide/1 -> Tgen/1

== system simli_gridSI/omega turbine to T_gen ==
  omega_WTR : Inport
  Constant : Constant  Value=P_aero_0
  Divide : Product  Inputs=**/
  Square : Math  Operator=square
  turbine omega operating point : Constant  Value=(omega_WTR_0/omega_WTR_n)
  Tgen : Outport
  wires:
  omega_WTR/1 -> Divide/1
  Divide/1 -> Tgen/1
  Constant/1 -> Divide/2
  turbine omega operating point/1 -> Square/1
  Square/1 -> Divide/3

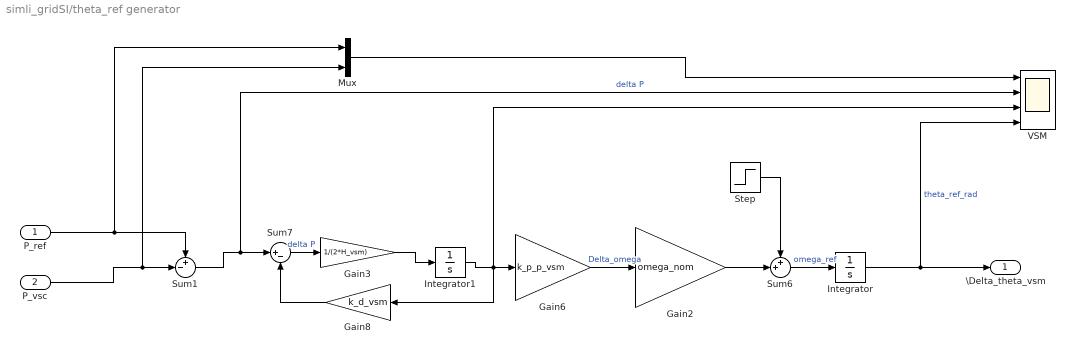
== system simli_gridSI/theta_ref generator ==
  P_ref : Inport
  P_vsc : Inport  Port=2
  Gain2 : Gain  Gain=omega_nom
  Gain3 : Gain  Gain=1/(2*H_vsm)
  Gain6 : Gain  Gain=k_p_p_vsm
  Gain8 : Gain  Gain=k_d_vsm
  Integrator : Integrator  WrappedStateUpperValue=2*pi  WrappedStateLowerValue=0
  Integrator1 : Integrator
  Mux : Mux  Inputs=2
  Step : Step  Time=5  After=0  SampleTime=Ts_power
  Sum1 : Sum  Inputs=+-|
  Sum6 : Sum  Inputs=++|
  Sum7 : Sum  Inputs=|+-
  VSM : Scope  NumInputPorts=4
  \Delta_theta_vsm : Outport
  wires:
  Gain3/1 -> Integrator1/1
  Sum1/1 -> VSM/2, Sum7/1  "delta P"
  Integrator1/1 -> VSM/3, Gain6/1, Gain8/1
  Gain8/1 -> Sum7/2
  Gain6/1 -> Gain2/1  "Delta_omega"
  Sum7/1 -> Gain3/1  "delta P"
  Gain2/1 -> Sum6/2
  P_ref/1 -> Mux/1, Sum1/1
  P_vsc/1 -> Mux/2, Sum1/2
  Integrator/1 -> VSM/4, \Delta_theta_vsm/1  "theta_ref_rad"
  Sum6/1 -> Integrator/1  "omega_ref"
  Step/1 -> Sum6/1
  Mux/1 -> VSM/1
